simulink library "chyc_rebuild_chyc_20170830_std"  (R2012b)
settings: Solver=ode45  StartTime=0.0  StopTime=10.0  RelTol=1e-3
undefined symbols (not defined in the file): sMP
libraries: simulink x6, simulink_extras x1
settings Model: Creator=LAUEREL  LastModifiedBy=LAUEREL

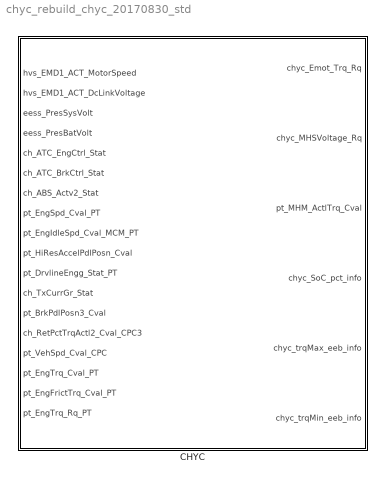
== system chyc_rebuild_chyc_20170830_std ==
  CHYC : Subsystem  mask(MapModule){chyc_EM_BstApp_DeltaEngSpd=sMP.ctrl.chyc.EM_BstApp_DeltaEngSpd, chyc_EM_BstApp_thresh_AccPedal=sMP.ctrl.chyc.EM_BstApp_thresh_AccPedal, chyc_EM_BstTrq_BrkPt_SoC=sMP.ctrl.chyc.EM_BstTrq_BrkPt_SoC, chyc_EM_BstTrq_BrkPt_VehSpd=sMP.ctrl.chyc.EM_BstTrq_BrkPt_VehSpd, chyc_EM_BstTrq_Map_BstTrq=sMP.ctrl.chyc.EM_BstTrq_Map_BstTrq, chyc_EM_BstTrq_TrqAuxSupport=sMP.ctrl.chyc.EM_BstTrq_TrqAuxSupport, chyc_EM_BstTrq_hyst_SoCforAuxSupport=sMP.ctrl.chyc.EM_BstTrq_hyst_SoCforAuxSupport, chyc_EM_BstTrq_thresh_GearforBoost=sMP.ctrl.chyc.EM_BstTrq_thresh_GearforBoost, chyc_EM_BstTrq_thresh_SoCforAuxSupport=sMP.ctrl.chyc.EM_BstTrq_thresh_SoCforAuxSupport, chyc_EM_ElBound_CurrMax=sMP.ctrl.chyc.EM_ElBound_CurrMax, chyc_EM_ElBound_CurrMin=sMP.ctrl.chyc.EM_ElBound_CurrMin, chyc_EM_ElBound_VltMax=sMP.ctrl.chyc.EM_ElBound_VltMax, chyc_EM_ElBound_VltMin=sMP.ctrl.chyc.EM_ElBound_VltMin, chyc_EM_ElBound_VltTarget=sMP.ctrl.chyc.EM_ElBound_VltTarget, chyc_EM_Fummel_TrqTargetLimit_boost=sMP.ctrl.chyc.EM_Fummel_TrqTargetLimit_boost, chyc_EM_Fummel_TrqTargetLimit_recup=sMP.ctrl.chyc.EM_Fummel_TrqTargetLimit_recup, chyc_EM_Fummel_rateDelay_ZeroCross_boost=sMP.ctrl.chyc.EM_Fummel_rateDelay_ZeroCross_boost, chyc_EM_Fummel_rateDelay_ZeroCross_recup=sMP.ctrl.chyc.EM_Fummel_rateDelay_ZeroCross_recup, chyc_EM_Fummel_trqRateLimit_ZeroCross_boost=sMP.ctrl.chyc.EM_Fummel_trqRateLimit_ZeroCross_boost, chyc_EM_Fummel_trqRateLimit_ZeroCross_recup=sMP.ctrl.chyc.EM_Fummel_trqRateLimit_ZeroCross_recup, chyc_EM_Fummel_trqRateLimit_boost=sMP.ctrl.chyc.EM_Fummel_trqRateLimit_boost, chyc_EM_Fummel_trqRateLimit_recup=sMP.ctrl.chyc.EM_Fummel_trqRateLimit_recup, chyc_EM_Fummel_trqThreshold_ZeroCross_boost=sMP.ctrl.chyc.EM_Fummel_trqThreshold_ZeroCross_boost, chyc_EM_Fummel_trqThreshold_ZeroCross_recup=sMP.ctrl.chyc.EM_Fummel_trqThreshold_ZeroCross_recup, chyc_EM_RecApp_thresh_GearforRecup=sMP.ctrl.chyc.EM_RecApp_thresh_GearforRecup, chyc_EM_RecApp_thresh_NoAccPedal=sMP.ctrl.chyc.EM_RecApp_thresh_NoAccPedal, chyc_EM_RecTrq_MaxRecTrq=sMP.ctrl.chyc.EM_RecTrq_MaxRecTrq, chyc_EM_RecTrq_PropFactor=sMP.ctrl.chyc.EM_RecTrq_PropFactor, chyc_EM_RecTrq_RWhl=sMP.ctrl.chyc.EM_RecTrq_RWhl, chyc_EM_RecTrq_RefWeight=sMP.ctrl.chyc.EM_RecTrq_RefWeight, chyc_EM_RecTrq_thresh_RetTrq=sMP.ctrl.chyc.EM_RecTrq_thresh_RetTrq, chyc_EM_TgtDet_EMTrqcutoff_abs=sMP.ctrl.chyc.EM_TgtDet_EMTrqcutoff_abs, chyc_EM_TgtDet_thresh_EngSpdAboveIdle=sMP.ctrl.chyc.EM_TgtDet_thresh_EngSpdAboveIdle, chyc_EM_TgtDet_thresh_EngTrqforRecup=sMP.ctrl.chyc.EM_TgtDet_thresh_EngTrqforRecup, chyc_EM_TgtDet_trqRateLimit_EBS_activate_neg=sMP.ctrl.chyc.EM_TgtDet_trqRateLimit_EBS_activate_neg, chyc_EM_TgtDet_trqRateLimit_EBS_activate_pos=sMP.ctrl.chyc.EM_TgtDet_trqRateLimit_EBS_activate_pos, chyc_EM_TgtDet_trqRateLimit_boost=sMP.ctrl.chyc.EM_TgtDet_trqRateLimit_boost, chyc_EM_TgtDet_trqRateLimit_recup=sMP.ctrl.chyc.EM_TgtDet_trqRateLimit_recup, chyc_EM_VersionNumber=sMP.ctrl.chyc.EM_VersionNumber, chyc_MHS_capacity=sMP.ctrl.chyc.MHS_capacity, chyc_MHS_U_cap_max=sMP.ctrl.chyc.MHS_U_cap_max, chyc_MHS_U_cap_min=sMP.ctrl.chyc.MHS_U_cap_min, chyc_MHS_nParallel=sMP.ctrl.chyc.MHS_nParallel, chyc_MHS_dcdc_Pmax_chg=sMP.ctrl.chyc.MHS_dcdc_Pmax_chg, chyc_MHS_dcdc_Pmax_dischg=sMP.ctrl.chyc.MHS_dcdc_Pmax_dischg, chyc_MHS_dcdc_U_Cap=sMP.ctrl.chyc.MHS_dcdc_U_Cap, chyc_MHS_dcdc_U_ZK=sMP.ctrl.chyc.MHS_dcdc_U_ZK, chyc_MHS_PEEBmax=sMP.ctrl.chyc.MHS_PEEBmax, chyc_mot_trqTab=sMP.ctrl.chyc.mot_trqTab, chyc_mot_nTab=sMP.ctrl.chyc.mot_nTab, chyc_mot_vltTab=sMP.ctrl.chyc.mot_vltTab, chyc_mot_Pmax_PTab=sMP.ctrl.chyc.mot_Pmax_PTab, chyc_mot_Pmax_PTab_trqTab=sMP.ctrl.chyc.mot_Pmax_PTab_trqTab, chyc_mot_eng_Pmax_HiLS=sMP.ctrl.chyc.mot_eng_Pmax_HiLS, chyc_mot_trqMax_vltTab=sMP.ctrl.chyc.mot_trqMax_vltTab, chyc_mot_trqMax_nTab=sMP.ctrl.chyc.mot_trqMax_nTab, chyc_mot_trqMax_trqTab_peak=sMP.ctrl.chyc.mot_trqMax_trqTab_peak, chyc_mot_trqMin_vltTab=sMP.ctrl.chyc.mot_trqMin_vltTab, chyc_mot_trqMin_nTab=sMP.ctrl.chyc.mot_trqMin_nTab, chyc_mot_trqMin_trqTab_peak=sMP.ctrl.chyc.mot_trqMin_trqTab_peak}

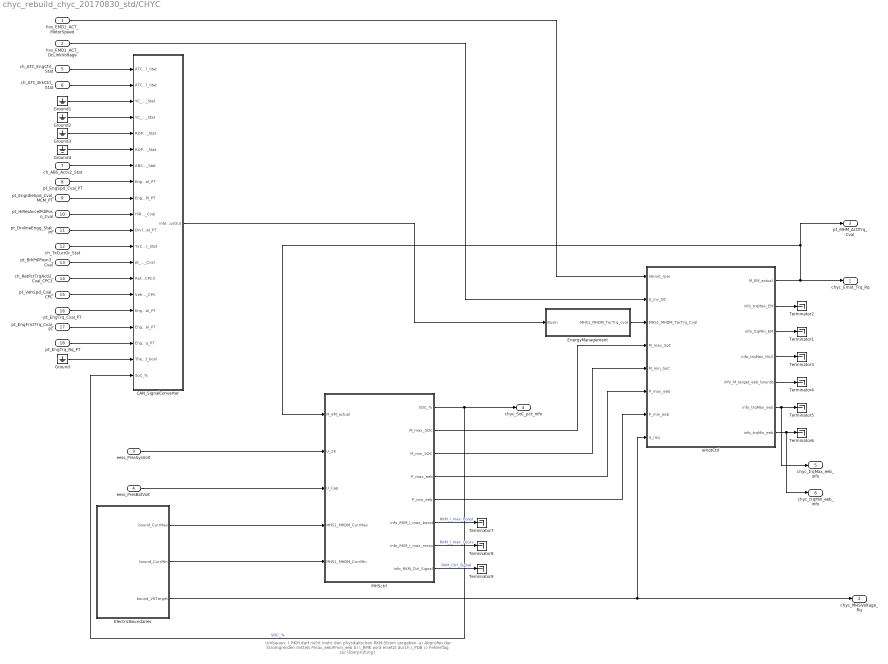
== system chyc_rebuild_chyc_20170830_std/CHYC ==
  note: Umbauen: I_RKM darf nicht mehr den physikalischen RKM-Strom vorgeben.
      | a) Abprüfen der Stromgrenzen mittels Pmax_eeb/Pmin_eeb
      | b) I_RMK wird ersetzt durch I_PDB
      | c) Fehlerflag zur Überprüfung?
  hvs_EMD1_ACT_MotorSpeed : Inport
  hvs_EMD1_ACT_DcLinkVoltage : Inport  Port=2
  eess_PresSysVolt : Inport  Port=3
  eess_PresBatVolt : Inport  Port=4
  ch_ATC_EngCtrl_Stat : Inport  Port=5
  ch_ATC_BrkCtrl_Stat : Inport  Port=6
  ch_ABS_Actv2_Stat : Inport  Port=7
  pt_EngSpd_Cval_PT : Inport  Port=8
  pt_EngIdleSpd_Cval_MCM_PT : Inport  Port=9
  pt_HiResAccelPdlPosn_Cval : Inport  Port=10
  pt_DrvlineEngg_Stat_PT : Inport  Port=11
  ch_TxCurrGr_Stat : Inport  Port=12
  pt_BrkPdlPosn3_Cval : Inport  Port=13
  ch_RetPctTrqActl2_Cval_CPC3 : Inport  Port=14
  pt_VehSpd_Cval_CPC : Inport  Port=15
  pt_EngTrq_Cval_PT : Inport  Port=16
  pt_EngFrictTrq_Cval_PT : Inport  Port=17
  pt_EngTrq_Rq_PT : Inport  Port=18
  CAN_SignalConverter : Subsystem
  ElectricBoundaries : Subsystem
  EnergyManagement : Subsystem
  Ground{,1..4} (5 alike) : Ground
  MHSctrl : Subsystem
  Terminator{1..9} (9 alike) : Terminator
  emotCtrl : Subsystem
  chyc_Emot_Trq_Rq : Outport
  chyc_MHSVoltage_Rq : Outport  Port=2
  pt_MHM_ActlTrq_Cval : Outport  Port=3
  chyc_SoC_pct_info : Outport  Port=4
  chyc_trqMax_eeb_info : Outport  Port=5
  chyc_trqMin_eeb_info : Outport  Port=6
  wires:
  EnergyManagement/1(MHS1_MHDM_TarTrq_cval) -> emotCtrl/3(MHS1_MHDM_TarTrq_Cval)
  CAN_SignalConverter/1(internalBusOut) -> EnergyManagement/1(BusIn)
  emotCtrl/2(info_trqMax_EM) -> Terminator2/1
  emotCtrl/3(info_trqMin_EM) -> Terminator1/1
  emotCtrl/4(info_trqMax_HiLS) -> Terminator3/1
  emotCtrl/5(info_M_target_eeb_bounds) -> Terminator4/1
  emotCtrl/6(info_trqMax_eeb) -> chyc_trqMax_eeb_info/1, Terminator5/1
  emotCtrl/7(info_trqMin_eeb) -> chyc_trqMin_eeb_info/1, Terminator6/1
  emotCtrl/1(M_EM_actual) -> chyc_Emot_Trq_Rq/1, pt_MHM_ActlTrq_Cval/1, MHSctrl/1(M_EM_actual)
  eess_PresSysVolt/1 -> MHSctrl/2(U_ZK)
  eess_PresBatVolt/1 -> MHSctrl/3(U_Cap)
  MHSctrl/3(M_min_SOC) -> emotCtrl/5(M_min_SoC)
  MHSctrl/2(M_max_SOC) -> emotCtrl/4(M_max_SoC)
  MHSctrl/1(SOC_%) -> CAN_SignalConverter/20(SoC_%), chyc_SoC_pct_info/1  "SOC_%"
  ElectricBoundaries/3(bound_VltTarget) -> chyc_MHSVoltage_Rq/1, emotCtrl/8(U_req)
  ElectricBoundaries/1(bound_CurrMax) -> MHSctrl/4(MHS1_MHDM_CurrMax)
  ElectricBoundaries/2(bound_CurrMin) -> MHSctrl/5(MHS1_MHDM_CurrMin)
  MHSctrl/6(info_RKM_I_max_boost) -> Terminator7/1  "RKM_I_max_boost"
  MHSctrl/7(info_RKM_I_max_recov) -> Terminator8/1  "RKM_I_max_recov"
  MHSctrl/8(info_RKM_Ctrl_Signal) -> Terminator9/1  "RKM_Ctrl_Signal"
  hvs_EMD1_ACT_MotorSpeed/1 -> emotCtrl/1(nEmot_rpm)
  MHSctrl/5(P_min_eeb) -> emotCtrl/7(P_min_eeb)
  MHSctrl/4(P_max_eeb) -> emotCtrl/6(P_max_eeb)
  hvs_EMD1_ACT_DcLinkVoltage/1 -> emotCtrl/2(U_inv_DC)
  Ground4/1 -> CAN_SignalConverter/6(ROP_EngCtrlActv2_Stat)
  pt_BrkPdlPosn3_Cval/1 -> CAN_SignalConverter/13(pt_BrkPdlPosn3_Cval)
  pt_EngTrq_Rq_PT/1 -> CAN_SignalConverter/18(EngTrqRq_PT)
  pt_EngSpd_Cval_PT/1 -> CAN_SignalConverter/8(EngSpd_Cval_PT)
  pt_HiResAccelPdlPosn_Cval/1 -> CAN_SignalConverter/10(HiResAccelPosn_Cval)
  pt_EngFrictTrq_Cval_PT/1 -> CAN_SignalConverter/17(EngFricTrq_Cval_PT)
  ch_ATC_BrkCtrl_Stat/1 -> CAN_SignalConverter/2(ATC_BrkCtrl_Stat)
  ch_ATC_EngCtrl_Stat/1 -> CAN_SignalConverter/1(ATC_EngCtrl_Stat)
  ch_RetPctTrqActl2_Cval_CPC3/1 -> CAN_SignalConverter/14(RetPctTrqActl2_Cval_CPC3)
  pt_VehSpd_Cval_CPC/1 -> CAN_SignalConverter/15(VehSpd_Cval_CPC)
  pt_EngTrq_Cval_PT/1 -> CAN_SignalConverter/16(EngTrq_Cval_PT)
  Ground3/1 -> CAN_SignalConverter/5(ROP_BrkCtrlActv2_Stat)
  ch_TxCurrGr_Stat/1 -> CAN_SignalConverter/12(TxCurrGr_Stat)
  ch_ABS_Actv2_Stat/1 -> CAN_SignalConverter/7(ABS_Actv_Stat)
  Ground2/1 -> CAN_SignalConverter/4(YC_EngCtrlActv2_Stat)
  Ground/1 -> CAN_SignalConverter/19(ThermoSupport_bool)
  pt_DrvlineEngg_Stat_PT/1 -> CAN_SignalConverter/11(DrvlineEngg_Stat_PT)
  pt_EngIdleSpd_Cval_MCM_PT/1 -> CAN_SignalConverter/9(EngIdleSpd_Cval_MCM_PT)
  Ground1/1 -> CAN_SignalConverter/3(YC_BrkCtrlActv2_Stat)

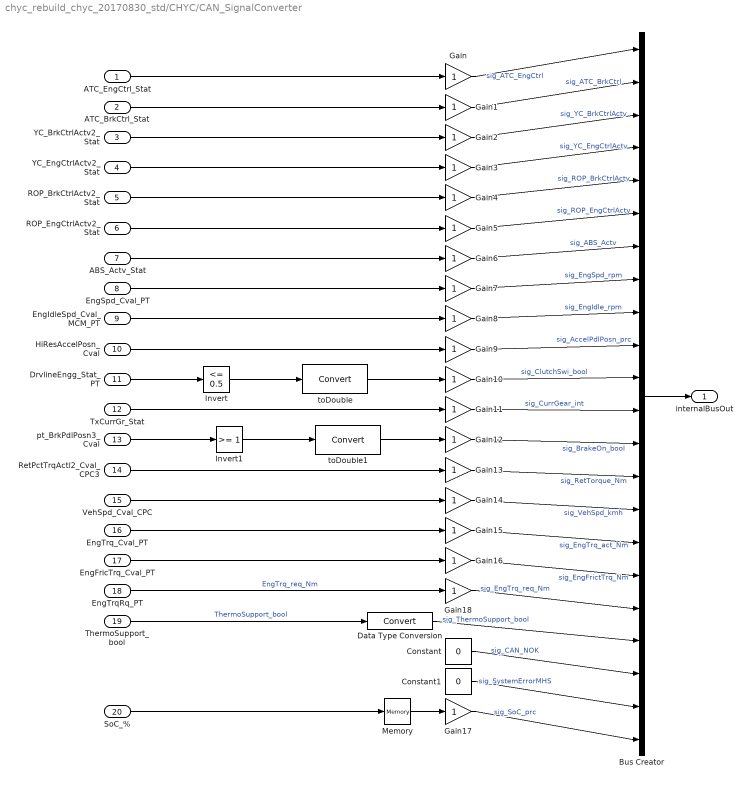
== system chyc_rebuild_chyc_20170830_std/CHYC/CAN_SignalConverter ==
  ATC_EngCtrl_Stat : Inport
  ATC_BrkCtrl_Stat : Inport  Port=2
  YC_BrkCtrlActv2_Stat : Inport  Port=3
  YC_EngCtrlActv2_Stat : Inport  Port=4
  ROP_BrkCtrlActv2_Stat : Inport  Port=5
  ROP_EngCtrlActv2_Stat : Inport  Port=6
  ABS_Actv_Stat : Inport  Port=7
  EngSpd_Cval_PT : Inport  Port=8
  EngIdleSpd_Cval_MCM_PT : Inport  Port=9
  HiResAccelPosn_Cval : Inport  Port=10
  DrvlineEngg_Stat_PT : Inport  Port=11
  TxCurrGr_Stat : Inport  Port=12
  pt_BrkPdlPosn3_Cval : Inport  Port=13
  RetPctTrqActl2_Cval_CPC3 : Inport  Port=14
  VehSpd_Cval_CPC : Inport  Port=15
  EngTrq_Cval_PT : Inport  Port=16
  EngFricTrq_Cval_PT : Inport  Port=17
  EngTrqRq_PT : Inport  Port=18
  ThermoSupport_bool : Inport  Port=19
  SoC_% : Inport  Port=20
  Bus Creator : BusCreator  Inputs=22
  Constant : Constant  Value=0
  Constant1 : Constant  Value=0
  Data Type Conversion : DataTypeConversion
  Gain{,1..18} (19 alike) : Gain
  Invert : simulink/Logic and Bit Operations/Compare To Constant  relop=<=  const=0.5  OutDataTypeStr=boolean
  Invert1 : simulink/Logic and Bit Operations/Compare To Constant  relop=>=  const=1  OutDataTypeStr=boolean
  Memory : Memory
  toDouble : DataTypeConversion
  toDouble1 : DataTypeConversion
  internalBusOut : Outport
  wires:
  SoC_%/1 -> Memory/1
  Gain/1 -> Bus Creator/1  "sig_ATC_EngCtrl"
  Gain1/1 -> Bus Creator/2  "sig_ATC_BrkCtrl"
  Gain2/1 -> Bus Creator/3  "sig_YC_BrkCtrlActv"
  Gain3/1 -> Bus Creator/4  "sig_YC_EngCtrlActv"
  Gain4/1 -> Bus Creator/5  "sig_ROP_BrkCtrlActv"
  Gain5/1 -> Bus Creator/6  "sig_ROP_EngCtrlActv"
  Gain9/1 -> Bus Creator/10  "sig_AccelPdlPosn_prc"
  Gain6/1 -> Bus Creator/7  "sig_ABS_Actv"
  Gain7/1 -> Bus Creator/8  "sig_EngSpd_rpm"
  Gain10/1 -> Bus Creator/11  "sig_ClutchSwi_bool"
  Gain8/1 -> Bus Creator/9  "sig_EngIdle_rpm"
  Gain11/1 -> Bus Creator/12  "sig_CurrGear_int"
  Gain12/1 -> Bus Creator/13  "sig_BrakeOn_bool"
  Gain13/1 -> Bus Creator/14  "sig_RetTorque_Nm"
  Gain15/1 -> Bus Creator/16  "sig_EngTrq_act_Nm"
  Gain14/1 -> Bus Creator/15  "sig_VehSpd_kmh"
  Gain17/1 -> Bus Creator/22  "sig_SoC_prc"
  Gain16/1 -> Bus Creator/17  "sig_EngFrictTrq_Nm"
  Data Type Conversion/1 -> Bus Creator/19  "sig_ThermoSupport_bool"
  Gain18/1 -> Bus Creator/18  "sig_EngTrq_req_Nm"
  Memory/1 -> Gain17/1
  Bus Creator/1 -> internalBusOut/1
  Constant/1 -> Bus Creator/20  "sig_CAN_NOK"
  Constant1/1 -> Bus Creator/21  "sig_SystemErrorMHS"
  TxCurrGr_Stat/1 -> Gain11/1
  EngFricTrq_Cval_PT/1 -> Gain16/1
  VehSpd_Cval_CPC/1 -> Gain14/1
  RetPctTrqActl2_Cval_CPC3/1 -> Gain13/1
  EngTrq_Cval_PT/1 -> Gain15/1
  Invert/1 -> toDouble/1
  HiResAccelPosn_Cval/1 -> Gain9/1
  EngIdleSpd_Cval_MCM_PT/1 -> Gain8/1
  ABS_Actv_Stat/1 -> Gain6/1
  ROP_EngCtrlActv2_Stat/1 -> Gain5/1
  ROP_BrkCtrlActv2_Stat/1 -> Gain4/1
  YC_EngCtrlActv2_Stat/1 -> Gain3/1
  YC_BrkCtrlActv2_Stat/1 -> Gain2/1
  ATC_BrkCtrl_Stat/1 -> Gain1/1
  ATC_EngCtrl_Stat/1 -> Gain/1
  EngSpd_Cval_PT/1 -> Gain7/1
  EngTrqRq_PT/1 -> Gain18/1  "EngTrq_req_Nm"
  ThermoSupport_bool/1 -> Data Type Conversion/1  "ThermoSupport_bool"
  DrvlineEngg_Stat_PT/1 -> Invert/1
  toDouble/1 -> Gain10/1
  Invert1/1 -> toDouble1/1
  toDouble1/1 -> Gain12/1
  pt_BrkPdlPosn3_Cval/1 -> Invert1/1

== system chyc_rebuild_chyc_20170830_std/CHYC/ElectricBoundaries ==
  CurrMax : Constant  Value=chyc_EM_ElBound_CurrMax
  CurrMin : Constant  Value=chyc_EM_ElBound_CurrMin
  VltTarget : Constant  Value=chyc_EM_ElBound_VltTarget
  bound_CurrMax : Outport
  bound_CurrMin : Outport  Port=2
  bound_VltTarget : Outport  Port=3
  wires:
  CurrMax/1 -> bound_CurrMax/1  "MHS1_MHDM_CurrMax_cval"
  CurrMin/1 -> bound_CurrMin/1  "MHS1_MHDM_CurrMin_cval"
  VltTarget/1 -> bound_VltTarget/1  "MHS1_MHDM_VltTarget"

== system chyc_rebuild_chyc_20170830_std/CHYC/EnergyManagement ==
  BusIn : Inport
  BoostApproval : Subsystem
  BoostTorque : Subsystem
  NoEBSFunction : Subsystem
  RecuperationApproval : Subsystem
  RecuperationTorque : Subsystem
  TargetDetermination : Subsystem
  MHS1_MHDM_TarTrq_cval : Outport
  wires:
  NoEBSFunction/1(NoEBSFunction) -> TargetDetermination/1(NoEBSFunction)
  TargetDetermination/1(MHS1_MHDM_TarTrq_cval) -> MHS1_MHDM_TarTrq_cval/1
  RecuperationApproval/1(RecApproved) -> TargetDetermination/2(RecApproved)
  BoostApproval/1(BoostApproved) -> TargetDetermination/3(BoostApproved)
  RecuperationTorque/1(TargetRecuperation) -> TargetDetermination/4(TargetRecuperation)
  BoostTorque/1(TargetBoost) -> TargetDetermination/5(TargetBoost)
  BusIn/1 -> BoostTorque/1(BusIn), TargetDetermination/6(BusIn), RecuperationTorque/1(BusIn), BoostApproval/1(BusIn), RecuperationApproval/1(BusIn), NoEBSFunction/1(BusIn)  "ClutchSwTop_Rq"

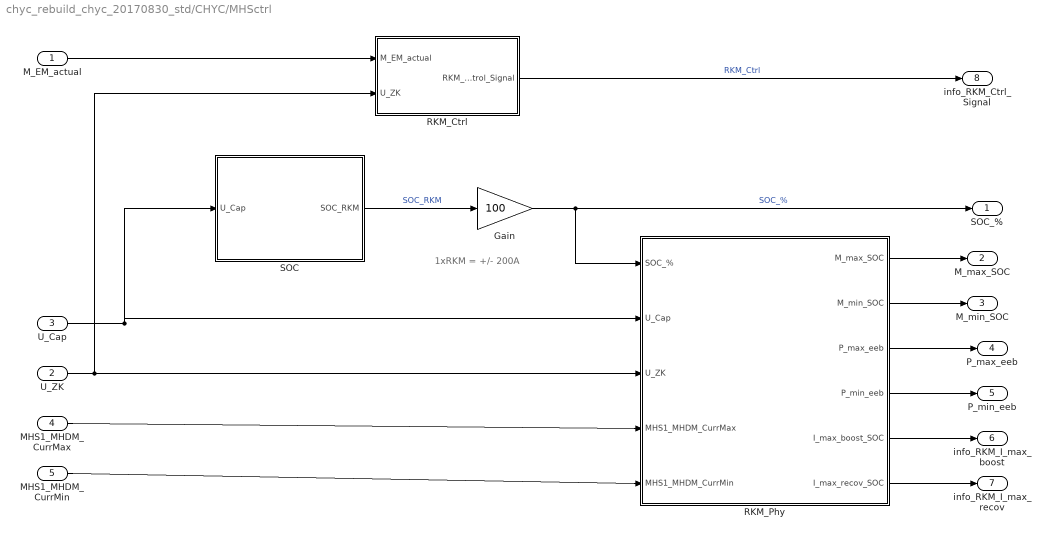
== system chyc_rebuild_chyc_20170830_std/CHYC/MHSctrl ==
  note: 1xRKM = +/- 200A
  M_EM_actual : Inport
  U_ZK : Inport  Port=2
  U_Cap : Inport  Port=3
  MHS1_MHDM_CurrMax : Inport  Port=4
  MHS1_MHDM_CurrMin : Inport  Port=5
  Gain : Gain  Gain=100
  "RKM_Ctrl " : Subsystem
  RKM_Phy : Subsystem
  SOC : Subsystem
  SOC_% : Outport  InitialOutput=0
  M_max_SOC : Outport  Port=2
  M_min_SOC : Outport  Port=3
  P_max_eeb : Outport  Port=4
  P_min_eeb : Outport  Port=5
  info_RKM_I_max_boost : Outport  Port=6
  info_RKM_I_max_recov : Outport  Port=7
  info_RKM_Ctrl_Signal : Outport  Port=8
  wires:
  RKM_Phy/4(P_min_eeb) -> P_min_eeb/1
  RKM_Phy/3(P_max_eeb) -> P_max_eeb/1
  RKM_Phy/2(M_min_SOC) -> M_min_SOC/1
  RKM_Phy/1(M_max_SOC) -> M_max_SOC/1
  RKM_Phy/6(I_max_recov_SOC) -> info_RKM_I_max_recov/1
  RKM_Phy/5(I_max_boost_SOC) -> info_RKM_I_max_boost/1
  Gain/1 -> RKM_Phy/1(SOC_%), SOC_%/1  "SOC_%"
  SOC/1(SOC_RKM) -> Gain/1  "SOC_RKM"
  U_Cap/1 -> SOC/1(U_Cap), RKM_Phy/2(U_Cap)
  U_ZK/1 -> RKM_Phy/3(U_ZK), "RKM_Ctrl "/2("U_ZK ")
  M_EM_actual/1 -> "RKM_Ctrl "/1(M_EM_actual)
  "RKM_Ctrl "/1(RKM_Control_Signal) -> info_RKM_Ctrl_Signal/1  "RKM_Ctrl"
  MHS1_MHDM_CurrMax/1 -> RKM_Phy/4(MHS1_MHDM_CurrMax)
  MHS1_MHDM_CurrMin/1 -> RKM_Phy/5(MHS1_MHDM_CurrMin)

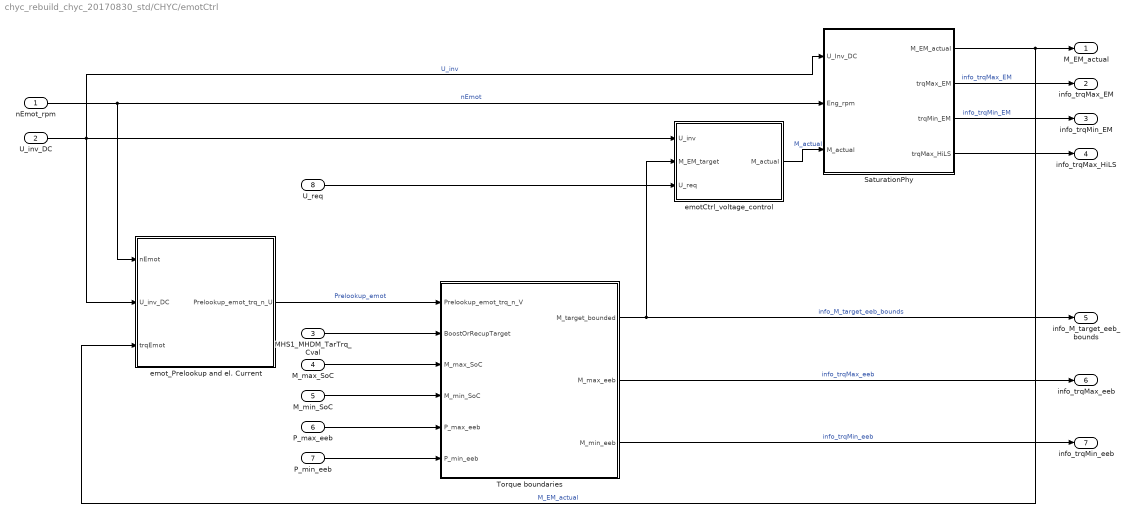
== system chyc_rebuild_chyc_20170830_std/CHYC/emotCtrl ==
  nEmot_rpm : Inport
  U_inv_DC : Inport  Port=2
  MHS1_MHDM_TarTrq_Cval : Inport  Port=3
  M_max_SoC : Inport  Port=4
  M_min_SoC : Inport  Port=5
  P_max_eeb : Inport  Port=6
  P_min_eeb : Inport  Port=7
  U_req : Inport  Port=8
  SaturationPhy : Subsystem
  Torque boundaries : Subsystem
  emotCtrl_voltage_control : Subsystem
  emot_Prelookup and el. Current : Subsystem
  M_EM_actual : Outport
  info_trqMax_EM : Outport  Port=2
  info_trqMin_EM : Outport  Port=3
  info_trqMax_HiLS : Outport  Port=4
  info_M_target_eeb_bounds : Outport  Port=5
  info_trqMax_eeb : Outport  Port=6
  info_trqMin_eeb : Outport  Port=7
  wires:
  SaturationPhy/1(M_EM_actual) -> emot_Prelookup and el. Current/3(trqEmot), M_EM_actual/1  "M_EM_actual"
  nEmot_rpm/1 -> emot_Prelookup and el. Current/1(nEmot), SaturationPhy/2(Eng_rpm)  "nEmot"
  U_inv_DC/1 -> emot_Prelookup and el. Current/2(U_inv_DC), SaturationPhy/1(U_Inv_DC), emotCtrl_voltage_control/1(U_inv)  "U_inv"
  MHS1_MHDM_TarTrq_Cval/1 -> Torque boundaries/2(BoostOrRecupTarget)
  emotCtrl_voltage_control/1(M_actual) -> SaturationPhy/3(M_actual)  "M_actual"
  SaturationPhy/2(trqMax_EM) -> info_trqMax_EM/1  "info_trqMax_EM"
  SaturationPhy/3(trqMin_EM) -> info_trqMin_EM/1  "info_trqMin_EM"
  SaturationPhy/4(trqMax_HiLS) -> info_trqMax_HiLS/1
  P_max_eeb/1 -> Torque boundaries/5(P_max_eeb)
  M_max_SoC/1 -> Torque boundaries/3(M_max_SoC)
  M_min_SoC/1 -> Torque boundaries/4(M_min_SoC)
  P_min_eeb/1 -> Torque boundaries/6(P_min_eeb)
  Torque boundaries/1(M_target_bounded) -> info_M_target_eeb_bounds/1, emotCtrl_voltage_control/2(M_EM_target)  "info_M_target_eeb_bounds"
  Torque boundaries/2(M_max_eeb) -> info_trqMax_eeb/1  "info_trqMax_eeb"
  Torque boundaries/3(M_min_eeb) -> info_trqMin_eeb/1  "info_trqMin_eeb"
  U_req/1 -> emotCtrl_voltage_control/3(U_req)
  emot_Prelookup and el. Current/1(Prelookup_emot_trq_n_U) -> Torque boundaries/1(Prelookup_emot_trq_n_V)  "Prelookup_emot"

== system chyc_rebuild_chyc_20170830_std/CHYC/EnergyManagement/BoostApproval ==
  BusIn : Inport
  Accpdl : RelationalOperator  Operator=>  OutDataTypeStr=boolean
  Add : Sum
  Bus Selector2 : BusSelector  OutputSignals=sig_ThermoSupport_bool,sig_AccelPdlPosn_prc,sig_EngSpd_rpm,sig_EngIdle_rpm
  Constant1 : Constant  Value=chyc_EM_BstApp_thresh_AccPedal  OutDataTypeStr=uint16
  Constant2 : Constant  Value=0  OutDataTypeStr=uint16
  Logical Operator : Logic  AllPortsSameDT=off  OutDataTypeStr=boolean
  Logical Operator1 : Logic  Operator=OR  AllPortsSameDT=off  OutDataTypeStr=boolean
  NoDriveoffPossible : RelationalOperator  Operator=<  OutDataTypeStr=boolean
  NoThermoSupport : RelationalOperator  Operator===  OutDataTypeStr=boolean
  offset rpm : Constant  Value=chyc_EM_BstApp_DeltaEngSpd
  BoostApproved : Outport
  wires:
  NoThermoSupport/1 -> Logical Operator/1  "sig_NoThermoSupport"
  Constant2/1 -> NoThermoSupport/2
  Accpdl/1 -> Logical Operator1/1
  Logical Operator1/1 -> Logical Operator/2  "sig_TractionStateOrIdle"
  Constant1/1 -> Accpdl/2
  Logical Operator/1 -> BoostApproved/1  "sig_BoostApproved"
  NoDriveoffPossible/1 -> Logical Operator1/2
  Add/1 -> NoDriveoffPossible/2
  offset rpm/1 -> Add/2
  Bus Selector2/4 -> Add/1  "<sig_EngIdle_rpm>"
  BusIn/1 -> Bus Selector2/1  "ClutchSwTop_Rq"
  Bus Selector2/3 -> NoDriveoffPossible/1  "<sig_EngSpd_rpm>"
  Bus Selector2/1 -> NoThermoSupport/1  "<sig_ThermoSupport_bool>"
  Bus Selector2/2 -> Accpdl/1  "<sig_AccelPdlPosn_prc>"

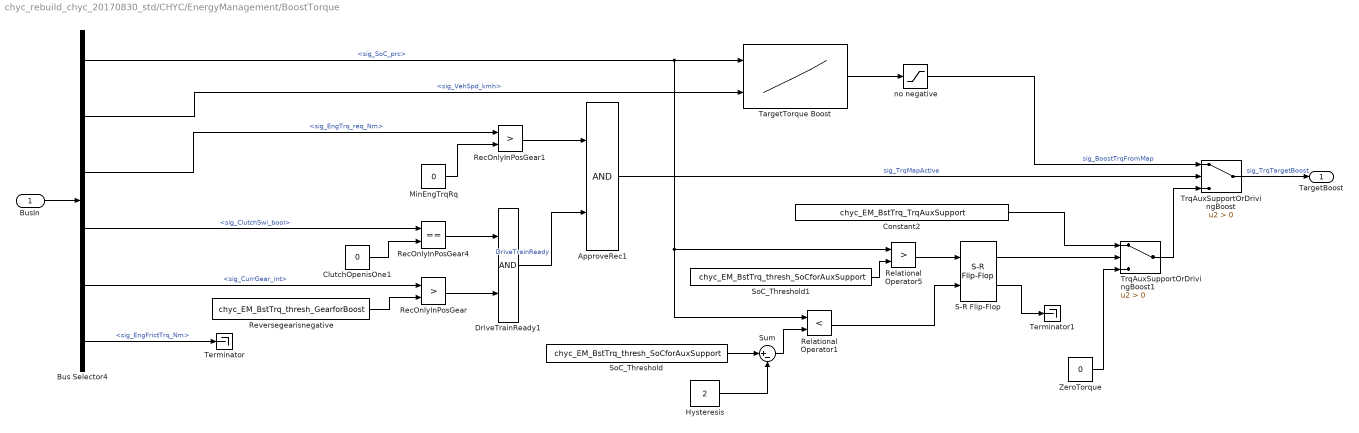
== system chyc_rebuild_chyc_20170830_std/CHYC/EnergyManagement/BoostTorque ==
  BusIn : Inport
  ApproveRec1 : Logic  AllPortsSameDT=off  OutDataTypeStr=boolean
  Bus Selector4 : BusSelector  OutputSignals=sig_SoC_prc,sig_VehSpd_kmh,sig_EngTrq_req_Nm,sig_ClutchSwi_bool,sig_CurrGear_int,sig_EngFrictTrq_Nm
  ClutchOpenisOne1 : Constant  Value=0
  Constant2 : Constant  Value=chyc_EM_BstTrq_TrqAuxSupport
  DriveTrainReady1 : Logic  AllPortsSameDT=off  OutDataTypeStr=boolean
  Hysteresis : Constant  Value=2
  MinEngTrqRq : Constant  Value=0
  RecOnlyInPosGear : RelationalOperator  Operator=>  OutDataTypeStr=boolean
  RecOnlyInPosGear1 : RelationalOperator  Operator=>  OutDataTypeStr=boolean
  RecOnlyInPosGear4 : RelationalOperator  Operator===  OutDataTypeStr=boolean
  Relational Operator1 : RelationalOperator  Operator=<  OutDataTypeStr=boolean
  Relational Operator5 : RelationalOperator  Operator=>  OutDataTypeStr=boolean
  Reversegearisnegative : Constant  Value=chyc_EM_BstTrq_thresh_GearforBoost  VectorParams1D=off
  S-R Flip-Flop : simulink_extras/Flip Flops/S-R Flip-Flop  initial_condition=0
  SoC_Threshold : Constant  Value=chyc_EM_BstTrq_thresh_SoCforAuxSupport
  SoC_Threshold1 : Constant  Value=chyc_EM_BstTrq_thresh_SoCforAuxSupport
  Sum : Sum  Inputs=|+-
  TargetTorque Boost : Lookup_n-D  BreakpointsForDimension1=chyc_EM_BstTrq_BrkPt_SoC  BreakpointsForDimension2=chyc_EM_BstTrq_BrkPt_VehSpd  Table=chyc_EM_BstTrq_Map_BstTrq  ExtrapMethod=Clip  UseLastTableValue=on  RndMeth=Simplest  InputSameDT=on
  Terminator : Terminator
  Terminator1 : Terminator
  TrqAuxSupportOrDrivingBoost : Switch  Criteria=u2 > Threshold
  TrqAuxSupportOrDrivingBoost1 : Switch  Criteria=u2 > Threshold
  ZeroTorque : Constant  Value=0
  no negative : Saturate  UpperLimit=inf  LowerLimit=0
  TargetBoost : Outport
  wires:
  TrqAuxSupportOrDrivingBoost1/1 -> TrqAuxSupportOrDrivingBoost/3
  ZeroTorque/1 -> TrqAuxSupportOrDrivingBoost1/3
  S-R Flip-Flop/2 -> Terminator1/1
  S-R Flip-Flop/1 -> TrqAuxSupportOrDrivingBoost1/2
  Relational Operator1/1 -> S-R Flip-Flop/2
  Sum/1 -> Relational Operator1/2
  Hysteresis/1 -> Sum/2
  SoC_Threshold/1 -> Sum/1
  RecOnlyInPosGear1/1 -> ApproveRec1/1
  no negative/1 -> TrqAuxSupportOrDrivingBoost/1  "sig_BoostTrqFromMap"
  TrqAuxSupportOrDrivingBoost/1 -> TargetBoost/1  "sig_TrqTargetBoost"
  SoC_Threshold1/1 -> Relational Operator5/2
  ApproveRec1/1 -> TrqAuxSupportOrDrivingBoost/2  "sig_TrqMapActive"
  TargetTorque Boost/1 -> no negative/1
  Constant2/1 -> TrqAuxSupportOrDrivingBoost1/1
  Relational Operator5/1 -> S-R Flip-Flop/1
  Reversegearisnegative/1 -> RecOnlyInPosGear/2
  RecOnlyInPosGear/1 -> DriveTrainReady1/2
  ClutchOpenisOne1/1 -> RecOnlyInPosGear4/2
  RecOnlyInPosGear4/1 -> DriveTrainReady1/1
  DriveTrainReady1/1 -> ApproveRec1/2  "DriveTrainReady"
  MinEngTrqRq/1 -> RecOnlyInPosGear1/2
  BusIn/1 -> Bus Selector4/1
  Bus Selector4/2 -> TargetTorque Boost/2  "<sig_VehSpd_kmh>"
  Bus Selector4/6 -> Terminator/1  "<sig_EngFrictTrq_Nm>"
  Bus Selector4/5 -> RecOnlyInPosGear/1  "<sig_CurrGear_int>"
  Bus Selector4/4 -> RecOnlyInPosGear4/1  "<sig_ClutchSwi_bool>"
  Bus Selector4/1 -> Relational Operator1/1, Relational Operator5/1, TargetTorque Boost/1  "<sig_SoC_prc>"
  Bus Selector4/3 -> RecOnlyInPosGear1/1  "<sig_EngTrq_req_Nm>"

== system chyc_rebuild_chyc_20170830_std/CHYC/EnergyManagement/NoEBSFunction ==
  BusIn : Inport
  ApproveRec : Logic  Operator=NOR  Inputs=9  AllPortsSameDT=off  OutDataTypeStr=boolean
  Bus Selector : BusSelector  OutputSignals=sig_ATC_EngCtrl,sig_ATC_BrkCtrl,sig_YC_BrkCtrlActv,sig_YC_EngCtrlActv,sig_ROP_BrkCtrlActv,sig_ROP_EngCtrlActv,sig_ABS_Actv,sig_CAN_NOK,sig_SystemErrorMHS
  NoEBSFunction : Outport
  wires:
  ApproveRec/1 -> NoEBSFunction/1  "sig_NoEBSFunction"
  Bus Selector/7 -> ApproveRec/7  "<sig_ABS_Actv>"
  Bus Selector/6 -> ApproveRec/6  "<sig_ROP_EngCtrlActv>"
  Bus Selector/5 -> ApproveRec/5  "<sig_ROP_BrkCtrlActv>"
  Bus Selector/4 -> ApproveRec/4  "<sig_YC_EngCtrlActv>"
  Bus Selector/1 -> ApproveRec/1  "<sig_ATC_EngCtrl>"
  Bus Selector/3 -> ApproveRec/3  "<sig_YC_BrkCtrlActv>"
  Bus Selector/2 -> ApproveRec/2  "<sig_ATC_BrkCtrl>"
  BusIn/1 -> Bus Selector/1  "ClutchSwTop_Rq"
  Bus Selector/8 -> ApproveRec/8  "<sig_CAN_NOK>"
  Bus Selector/9 -> ApproveRec/9  "<sig_SystemErrorMHS>"

== system chyc_rebuild_chyc_20170830_std/CHYC/EnergyManagement/RecuperationApproval ==
  BusIn : Inport
  ApproveRec : Logic  AllPortsSameDT=off  OutDataTypeStr=boolean
  Bus Selector1 : BusSelector  OutputSignals=sig_AccelPdlPosn_prc,sig_ClutchSwi_bool,sig_CurrGear_int
  ClutchNotOpen : RelationalOperator  Operator===  OutDataTypeStr=boolean
  ClutchOpenisOne : Constant  Value=0
  DriveTrainReady : Logic  AllPortsSameDT=off  OutDataTypeStr=boolean
  No AccPedal : RelationalOperator  Operator===  OutDataTypeStr=boolean
  RecOnlyInPosGear : RelationalOperator  Operator=>  OutDataTypeStr=boolean
  Reversegearisnegative : Constant  Value=chyc_EM_RecApp_thresh_GearforRecup
  par_EM_RecApp_thresh_NoAccPedal : Constant  Value=chyc_EM_RecApp_thresh_NoAccPedal
  RecApproved : Outport
  wires:
  Reversegearisnegative/1 -> RecOnlyInPosGear/2
  RecOnlyInPosGear/1 -> DriveTrainReady/2
  Bus Selector1/2 -> ClutchNotOpen/1  "<sig_ClutchSwi_bool>"
  ApproveRec/1 -> RecApproved/1  "sig_RecApproved"
  Bus Selector1/1 -> No AccPedal/1  "<sig_AccelPdlPosn_prc>"
  par_EM_RecApp_thresh_NoAccPedal/1 -> No AccPedal/2
  No AccPedal/1 -> ApproveRec/1  "NoAccPdl"
  ClutchOpenisOne/1 -> ClutchNotOpen/2
  ClutchNotOpen/1 -> DriveTrainReady/1
  DriveTrainReady/1 -> ApproveRec/2  "sig_DriveTrainReady"
  BusIn/1 -> Bus Selector1/1
  Bus Selector1/3 -> RecOnlyInPosGear/1  "<sig_CurrGear_int>"

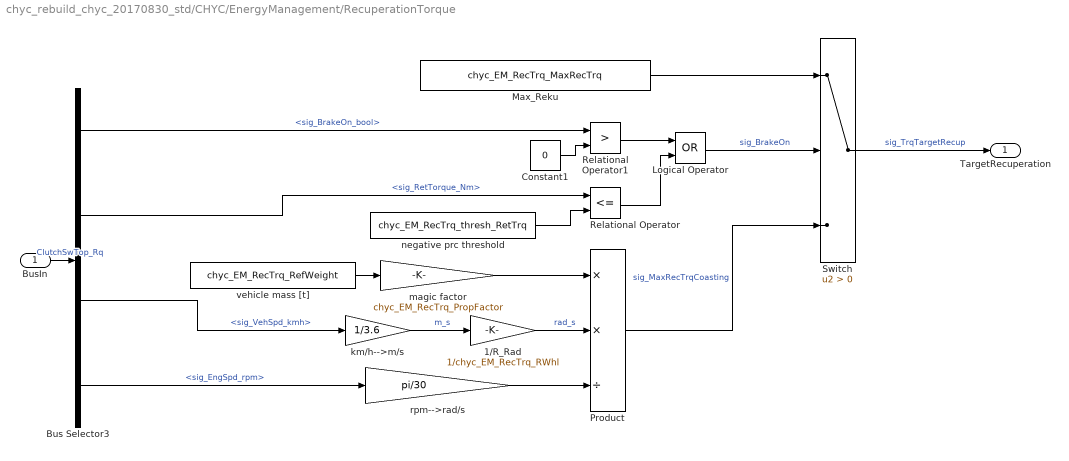
== system chyc_rebuild_chyc_20170830_std/CHYC/EnergyManagement/RecuperationTorque ==
  BusIn : Inport
  1/R_Rad : Gain  Gain=1/chyc_EM_RecTrq_RWhl
  Bus Selector3 : BusSelector  OutputSignals=sig_BrakeOn_bool,sig_RetTorque_Nm,sig_VehSpd_kmh,sig_EngSpd_rpm
  Constant1 : Constant  Value=0
  Logical Operator : Logic  Operator=OR  AllPortsSameDT=off  OutDataTypeStr=boolean
  Max_Reku : Constant  Value=chyc_EM_RecTrq_MaxRecTrq
  Product : Product  Inputs=**/  RndMeth=Zero
  Relational Operator : RelationalOperator  Operator=<=  OutDataTypeStr=boolean
  Relational Operator1 : RelationalOperator  Operator=>  OutDataTypeStr=boolean
  Switch : Switch  Criteria=u2 > Threshold
  km/h-->m/s : Gain  Gain=1/3.6
  magic factor : Gain  Gain=chyc_EM_RecTrq_PropFactor
  negative prc threshold : Constant  Value=chyc_EM_RecTrq_thresh_RetTrq
  rpm-->rad/s : Gain  Gain=pi/30
  vehicle mass [t] : Constant  Value=chyc_EM_RecTrq_RefWeight
  TargetRecuperation : Outport
  wires:
  magic factor/1 -> Product/1
  Constant1/1 -> Relational Operator1/2
  Relational Operator/1 -> Logical Operator/2
  negative prc threshold/1 -> Relational Operator/2
  Relational Operator1/1 -> Logical Operator/1
  Logical Operator/1 -> Switch/2  "sig_BrakeOn"
  Max_Reku/1 -> Switch/1
  Switch/1 -> TargetRecuperation/1  "sig_TrqTargetRecup"
  Product/1 -> Switch/3  "sig_MaxRecTrqCoasting"
  km/h-->m/s/1 -> 1/R_Rad/1  "m_s"
  1/R_Rad/1 -> Product/2  "rad_s"
  vehicle mass [t]/1 -> magic factor/1
  rpm-->rad/s/1 -> Product/3
  BusIn/1 -> Bus Selector3/1  "ClutchSwTop_Rq"
  Bus Selector3/1 -> Relational Operator1/1  "<sig_BrakeOn_bool>"
  Bus Selector3/2 -> Relational Operator/1  "<sig_RetTorque_Nm>"
  Bus Selector3/4 -> rpm-->rad/s/1  "<sig_EngSpd_rpm>"
  Bus Selector3/3 -> km/h-->m/s/1  "<sig_VehSpd_kmh>"

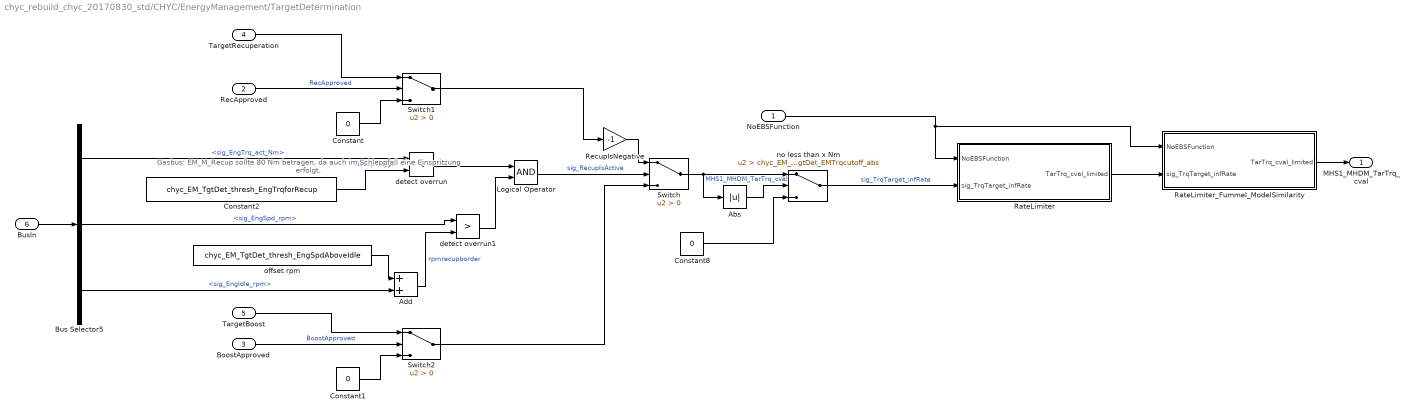
== system chyc_rebuild_chyc_20170830_std/CHYC/EnergyManagement/TargetDetermination ==
  note: Gasbus: EM_M_Recup sollte 80 Nm betragen, da auch im Schleppfall eine Einspritzung erfolgt.
  NoEBSFunction : Inport
  RecApproved : Inport  Port=2
  BoostApproved : Inport  Port=3
  TargetRecuperation : Inport  Port=4
  TargetBoost : Inport  Port=5
  BusIn : Inport  Port=6
  Abs : Abs
  Add : Sum
  Bus Selector5 : BusSelector  OutputSignals=sig_EngTrq_act_Nm,sig_EngSpd_rpm,sig_EngIdle_rpm
  Constant : Constant  Value=0
  Constant1 : Constant  Value=0
  Constant2 : Constant  Value=chyc_EM_TgtDet_thresh_EngTrqforRecup
  Constant8 : Constant  Value=0
  Logical Operator : Logic  AllPortsSameDT=off  OutDataTypeStr=boolean
  RateLimiter : Subsystem
  RateLimiter_Fummel_ModelSimilarity : Subsystem
  RecupIsNegative : Gain  Gain=-1
  Switch : Switch  Criteria=u2 > Threshold
  Switch1 : Switch  Criteria=u2 > Threshold
  Switch2 : Switch  Criteria=u2 > Threshold
  detect overrun : RelationalOperator  Operator=<  OutDataTypeStr=boolean
  detect overrun1 : RelationalOperator  Operator=>  OutDataTypeStr=boolean
  no less than x Nm : Switch  Criteria=u2 > Threshold  Threshold=chyc_EM_TgtDet_EMTrqcutoff_abs
  offset rpm : Constant  Value=chyc_EM_TgtDet_thresh_EngSpdAboveIdle
  MHS1_MHDM_TarTrq_cval : Outport
  wires:
  RateLimiter/1(TarTrq_cval_limited) -> RateLimiter_Fummel_ModelSimilarity/2(sig_TrqTarget_infRate)
  Abs/1 -> no less than x Nm/2
  Constant8/1 -> no less than x Nm/3
  Switch/1 -> no less than x Nm/1, Abs/1  "MHS1_MHDM_TarTrq_cval"
  RecApproved/1 -> Switch1/2  "RecApproved"
  BoostApproved/1 -> Switch2/2  "BoostApproved"
  Constant2/1 -> detect overrun/2  "RecupTrigger"
  TargetRecuperation/1 -> Switch1/1
  Constant/1 -> Switch1/3
  Switch1/1 -> RecupIsNegative/1
  TargetBoost/1 -> Switch2/1
  Constant1/1 -> Switch2/3
  Switch2/1 -> Switch/3
  detect overrun/1 -> Logical Operator/1
  detect overrun1/1 -> Logical Operator/2
  Add/1 -> detect overrun1/2  "rpmrecupborder"
  offset rpm/1 -> Add/1
  Logical Operator/1 -> Switch/2  "sig_RecupIsActive"
  RecupIsNegative/1 -> Switch/1
  Bus Selector5/1 -> detect overrun/1  "<sig_EngTrq_act_Nm>"
  Bus Selector5/2 -> detect overrun1/1  "<sig_EngSpd_rpm>"
  Bus Selector5/3 -> Add/2  "<sig_EngIdle_rpm>"
  BusIn/1 -> Bus Selector5/1
  NoEBSFunction/1 -> RateLimiter/1(NoEBSFunction), RateLimiter_Fummel_ModelSimilarity/1(NoEBSFunction)
  no less than x Nm/1 -> RateLimiter/2(sig_TrqTarget_infRate)  "sig_TrqTarget_infRate"
  RateLimiter_Fummel_ModelSimilarity/1(TarTrq_cval_limited) -> MHS1_MHDM_TarTrq_cval/1

== system chyc_rebuild_chyc_20170830_std/CHYC/MHSctrl/RKM_Ctrl  ==
  note: mit Logik für Recov / Boost
      | Recov:   RKM_C_S =
      | Boost:    RKM_C_S =
  M_EM_actual : Inport
  "U_ZK " : Inport  Port=2
  Logical Operator : Logic  AllPortsSameDT=off  OutDataTypeStr=boolean
  M_min : Constant  Value=0
  M_min1 : Constant  Value=51.8
  Relational Operator1 : RelationalOperator  Operator=>  OutDataTypeStr=boolean
  Relational Operator3 : RelationalOperator  Operator=<  OutDataTypeStr=boolean
  RKM_Control_Signal : Outport
  wires:
  Relational Operator3/1 -> Logical Operator/1
  Logical Operator/1 -> RKM_Control_Signal/1
  M_min/1 -> Relational Operator3/2
  M_min1/1 -> Relational Operator1/2
  "U_ZK "/1 -> Relational Operator1/1
  Relational Operator1/1 -> Logical Operator/2
  M_EM_actual/1 -> Relational Operator3/1

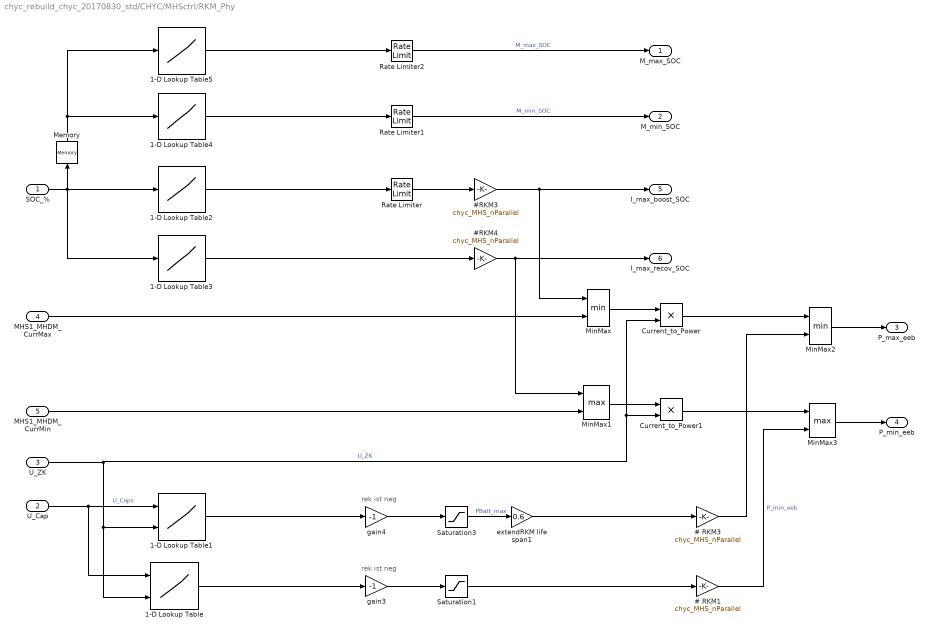
== system chyc_rebuild_chyc_20170830_std/CHYC/MHSctrl/RKM_Phy ==
  note: rek ist neg
  note: rek ist neg
  SOC_% : Inport
  U_Cap : Inport  Port=2
  U_ZK : Inport  Port=3
  MHS1_MHDM_CurrMax : Inport  Port=4
  MHS1_MHDM_CurrMin : Inport  Port=5
  # RKM1 : Gain  Gain=chyc_MHS_nParallel
  # RKM3 : Gain  Gain=chyc_MHS_nParallel
  #RKM3 : Gain  Gain=chyc_MHS_nParallel
  #RKM4 : Gain  Gain=chyc_MHS_nParallel
  1-D Lookup Table : Lookup_n-D  BreakpointsForDimension1=chyc_MHS_dcdc_U_Cap  BreakpointsForDimension2=chyc_MHS_dcdc_U_ZK  Table=chyc_MHS_dcdc_Pmax_chg  RndMeth=Simplest  InputSameDT=on
      settings: AttributesFormatString=%<Table>
  1-D Lookup Table1 : Lookup_n-D  BreakpointsForDimension1=chyc_MHS_dcdc_U_Cap  BreakpointsForDimension2=chyc_MHS_dcdc_U_ZK  Table=chyc_MHS_dcdc_Pmax_dischg  RndMeth=Simplest  InputSameDT=on
      settings: AttributesFormatString=%<Table>
  1-D Lookup Table2 : Lookup_n-D  NumberOfTableDimensions=1  BreakpointsForDimension1=[0,0.25,0.5,1,100]  Table=[0,20,80,200,200]  ExtrapMethod=Clip  UseLastTableValue=on  RndMeth=Simplest  InputSameDT=on
  1-D Lookup Table3 : Lookup_n-D  NumberOfTableDimensions=1  BreakpointsForDimension1=[0,99,99.5,99.75,100]  Table=[-200,-200,-80,-20,0]  ExtrapMethod=Clip  UseLastTableValue=on  RndMeth=Simplest  InputSameDT=on
  1-D Lookup Table4 : Lookup_n-D  NumberOfTableDimensions=1  BreakpointsForDimension1=[0,97,97.5,98,98.5,99,99.75,100]  Table=[-310,-310,-180,-50,-15,-5,-1,0]  ExtrapMethod=Clip  UseLastTableValue=on  RndMeth=Simplest  InputSameDT=on
  1-D Lookup Table5 : Lookup_n-D  NumberOfTableDimensions=1  BreakpointsForDimension1=[0,0.25,1,1.5,2,2.5,3,100]  Table=[0,1,5,15,50,180,310,310]  ExtrapMethod=Clip  UseLastTableValue=on  RndMeth=Simplest  InputSameDT=on
  Current_to_Power : Product  Inputs=**  RndMeth=Zero
  Current_to_Power1 : Product  Inputs=**  RndMeth=Zero
  Memory : Memory
  MinMax : MinMax  Inputs=2
  MinMax1 : MinMax  Function=max  Inputs=2
  MinMax2 : MinMax  Inputs=2
  MinMax3 : MinMax  Function=max  Inputs=2
  Rate Limiter : RateLimiter  RisingSlewLimit=200  FallingSlewLimit=-inf  SampleTimeMode=inherited
  Rate Limiter1 : RateLimiter  RisingSlewLimit=inf  FallingSlewLimit=-200  SampleTimeMode=inherited
  Rate Limiter2 : RateLimiter  RisingSlewLimit=200  FallingSlewLimit=-inf  SampleTimeMode=inherited
  Saturation1 : Saturate  UpperLimit=chyc_MHS_PEEBmax  LowerLimit=-chyc_MHS_PEEBmax
  Saturation3 : Saturate  UpperLimit=chyc_MHS_PEEBmax  LowerLimit=-chyc_MHS_PEEBmax
  extendRKM life span1 : Gain  Gain=0.6
  gain3 : Gain  Gain=-1
  gain4 : Gain  Gain=-1
  M_max_SOC : Outport
  M_min_SOC : Outport  Port=2
  P_max_eeb : Outport  Port=3
  P_min_eeb : Outport  Port=4
  I_max_boost_SOC : Outport  Port=5
  I_max_recov_SOC : Outport  Port=6
  wires:
  Memory/1 -> 1-D Lookup Table4/1, 1-D Lookup Table5/1
  1-D Lookup Table5/1 -> Rate Limiter2/1
  1-D Lookup Table4/1 -> Rate Limiter1/1
  Rate Limiter1/1 -> M_min_SOC/1  "M_min_SOC"
  Rate Limiter2/1 -> M_max_SOC/1  "M_max_SOC"
  1-D Lookup Table/1 -> gain3/1
  1-D Lookup Table1/1 -> gain4/1
  # RKM1/1 -> MinMax3/2  "P_min_eeb"
  # RKM3/1 -> MinMax2/2
  gain3/1 -> Saturation1/1
  gain4/1 -> Saturation3/1
  Saturation3/1 -> extendRKM life span1/1  "PBatt_max"
  1-D Lookup Table2/1 -> Rate Limiter/1
  U_ZK/1 -> Current_to_Power/2, Current_to_Power1/2, 1-D Lookup Table/2, 1-D Lookup Table1/2  "U_ZK"
  U_Cap/1 -> 1-D Lookup Table/1, 1-D Lookup Table1/1  "U_Caps"
  Rate Limiter/1 -> #RKM3/1
  #RKM3/1 -> MinMax/1, I_max_boost_SOC/1
  #RKM4/1 -> MinMax1/1, I_max_recov_SOC/1
  extendRKM life span1/1 -> # RKM3/1
  1-D Lookup Table3/1 -> #RKM4/1
  MHS1_MHDM_CurrMin/1 -> MinMax1/2
  SOC_%/1 -> Memory/1, 1-D Lookup Table3/1, 1-D Lookup Table2/1
  MHS1_MHDM_CurrMax/1 -> MinMax/2
  MinMax/1 -> Current_to_Power/1
  MinMax1/1 -> Current_to_Power1/1
  Current_to_Power/1 -> MinMax2/1
  Current_to_Power1/1 -> MinMax3/1
  MinMax2/1 -> P_max_eeb/1
  MinMax3/1 -> P_min_eeb/1
  Saturation1/1 -> # RKM1/1

== system chyc_rebuild_chyc_20170830_std/CHYC/MHSctrl/SOC ==
  note: SOC
  note: Ist_Energie
  note: Min_Energie
  note: E = 1/2 * C * (Umax^2 - Umin^2)
  U_Cap : Inport
  1/1 : Gain  Gain=1/2
  1/2 : Gain  Gain=1/2
  1/3 : Gain  Gain=1/2
  Add2 : Sum  Inputs=+-
  Add4 : Sum  Inputs=-+
  C : Gain  Gain=chyc_MHS_capacity
  "C " : Gain  Gain=chyc_MHS_capacity
  "C  " : Gain  Gain=chyc_MHS_capacity
  Divide1 : Product  Inputs=**
  Divide2 : Product  Inputs=**
  Divide3 : Product  Inputs=*/
  Divide4 : Product  Inputs=**
  U_cap_max : Constant  Value=chyc_MHS_U_cap_max
  U_cap_min : Constant  Value=chyc_MHS_U_cap_min
  SOC_RKM : Outport
  wires:
  U_Cap/1 -> Divide2/1, Divide2/2
  1/2/1 -> C/1
  Divide2/1 -> 1/2/1  "U_cap_quad"
  C/1 -> Add2/1
  1/1/1 -> "C "/1
  Divide1/1 -> 1/1/1  "U_cap_min_quad"
  U_cap_min/1 -> Divide1/2, Divide1/1
  "C "/1 -> Add2/2, Add4/1
  U_cap_max/1 -> Divide4/1, Divide4/2
  1/3/1 -> "C  "/1
  Divide4/1 -> 1/3/1  "U_cap_max_quad"
  "C  "/1 -> Add4/2
  Add2/1 -> Divide3/1  "E_delta_IST"
  Add4/1 -> Divide3/2  "E_delta_MAX"
  Divide3/1 -> SOC_RKM/1  "SOC_RKM"

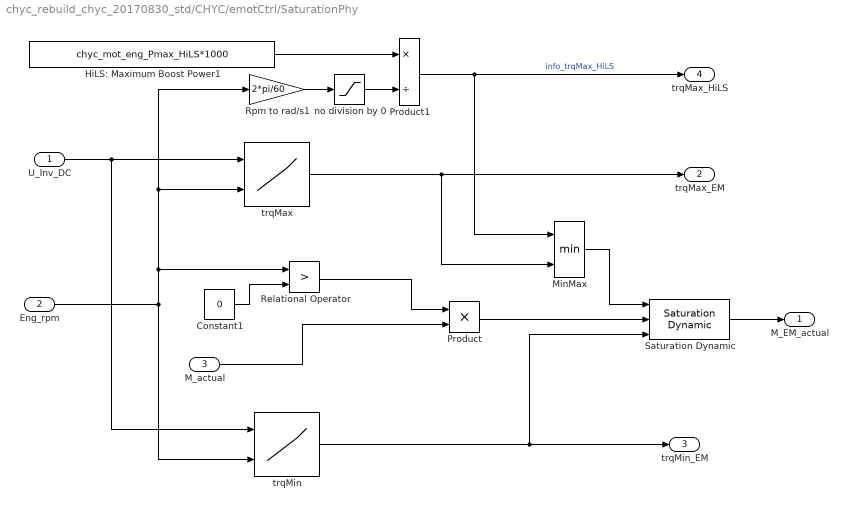
== system chyc_rebuild_chyc_20170830_std/CHYC/emotCtrl/SaturationPhy ==
  U_Inv_DC : Inport
  Eng_rpm : Inport  Port=2
  M_actual : Inport  Port=3
  Constant1 : Constant  Value=0
  HiLS: Maximum Boost Power1 : Constant  Value=chyc_mot_eng_Pmax_HiLS*1000
  MinMax : MinMax  Inputs=2
  Product : Product  RndMeth=Zero
  Product1 : Product  Inputs=*/  RndMeth=Zero
  Relational Operator : RelationalOperator  Operator=>  OutDataTypeStr=boolean
  Rpm to rad/s1 : Gain  Gain=2*pi/60
  Saturation Dynamic : simulink/Discontinuities/Saturation Dynamic  OutMin=[]  OutMax=[]  OutDataTypeStr=Inherit: Same as second input  OutDataType=fixdt(1, 16)  OutScaling=2^-10  DoSatur=off
  no division by 0 : Saturate  UpperLimit=inf  LowerLimit=10
  trqMax : Lookup_n-D  BreakpointsForDimension1=chyc_mot_trqMax_vltTab  BreakpointsForDimension2=chyc_mot_trqMax_nTab  BreakpointsForDimension3=[5, 7]  Table=chyc_mot_trqMax_trqTab_peak  RndMeth=Simplest  InputSameDT=on
  trqMin : Lookup_n-D  BreakpointsForDimension1=chyc_mot_trqMin_vltTab  BreakpointsForDimension2=chyc_mot_trqMin_nTab  BreakpointsForDimension3=[5, 7]  Table=chyc_mot_trqMin_trqTab_peak  RndMeth=Simplest  InputSameDT=on
  M_EM_actual : Outport
  trqMax_EM : Outport  Port=2
  trqMin_EM : Outport  Port=3
  trqMax_HiLS : Outport  Port=4
  wires:
  Constant1/1 -> Relational Operator/2
  Relational Operator/1 -> Product/1
  M_actual/1 -> Product/2
  Saturation Dynamic/1 -> M_EM_actual/1
  trqMin/1 -> trqMin_EM/1, Saturation Dynamic/3
  trqMax/1 -> trqMax_EM/1, MinMax/2
  Eng_rpm/1 -> trqMin/2, Rpm to rad/s1/1, trqMax/2, Relational Operator/1
  Product/1 -> Saturation Dynamic/2
  Product1/1 -> trqMax_HiLS/1, MinMax/1  "info_trqMax_HiLS"
  Rpm to rad/s1/1 -> no division by 0/1
  HiLS: Maximum Boost Power1/1 -> Product1/1
  MinMax/1 -> Saturation Dynamic/1
  U_Inv_DC/1 -> trqMin/1, trqMax/1
  no division by 0/1 -> Product1/2

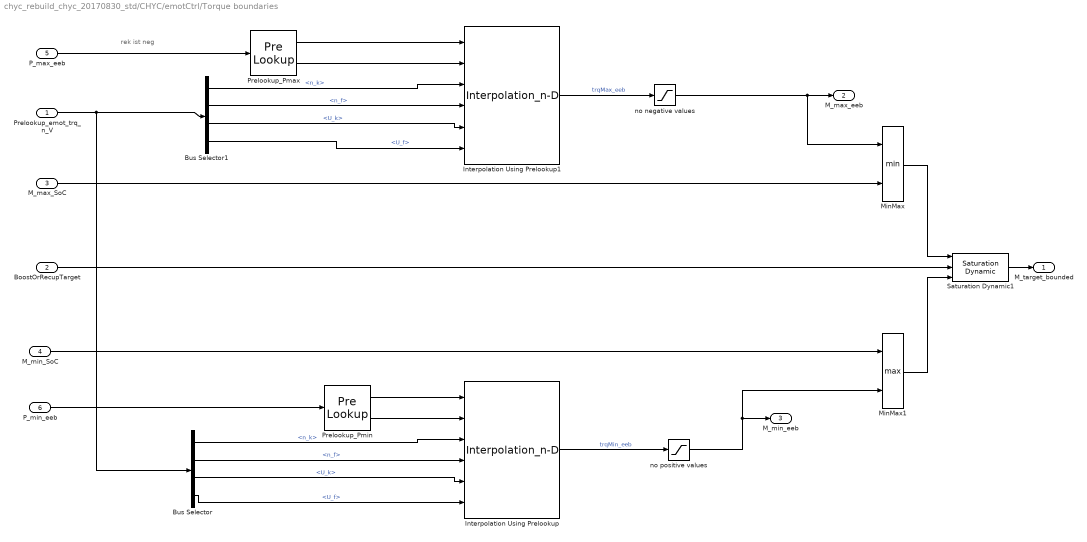
== system chyc_rebuild_chyc_20170830_std/CHYC/emotCtrl/Torque boundaries ==
  note: rek ist neg
  Prelookup_emot_trq_n_V : Inport
  BoostOrRecupTarget : Inport  Port=2
  M_max_SoC : Inport  Port=3
  M_min_SoC : Inport  Port=4
  P_max_eeb : Inport  Port=5
  P_min_eeb : Inport  Port=6
  Bus Selector : BusSelector  OutputSignals=n_k,n_f,U_k,U_f
  Bus Selector1 : BusSelector  OutputSignals=n_k,n_f,U_k,U_f
  Interpolation Using Prelookup : Interpolation_n-D  NumberOfTableDimensions=3  Table=chyc_mot_Pmax_PTab_trqTab
      settings: InputPortMap=u0,u1,u2,u3,u4,u5
  Interpolation Using Prelookup1 : Interpolation_n-D  NumberOfTableDimensions=3  Table=chyc_mot_Pmax_PTab_trqTab
      settings: InputPortMap=u0,u1,u2,u3,u4,u5
  MinMax : MinMax  Inputs=2
  MinMax1 : MinMax  Function=max  Inputs=2
  Prelookup_Pmax : PreLookup  BreakpointsData=chyc_mot_Pmax_PTab  IndexSearchMethod=Linear search  BeginIndexSearchUsingPreviousIndexResult=on  ExtrapMethod=Linear
  Prelookup_Pmin : PreLookup  BreakpointsData=chyc_mot_Pmax_PTab  IndexSearchMethod=Linear search  BeginIndexSearchUsingPreviousIndexResult=on  ExtrapMethod=Linear
  Saturation Dynamic1 : simulink/Discontinuities/Saturation Dynamic  OutMin=[]  OutMax=[]  OutDataTypeStr=Inherit: Same as second input  OutDataType=fixdt(1, 16)  OutScaling=2^-10  DoSatur=off
  no negative values : Saturate  UpperLimit=inf  LowerLimit=0
  no positive values : Saturate  UpperLimit=0  LowerLimit=-inf
  M_target_bounded : Outport
  M_max_eeb : Outport  Port=2
  M_min_eeb : Outport  Port=3
  wires:
  Interpolation Using Prelookup/1 -> no positive values/1  "trqMin_eeb"
  Interpolation Using Prelookup1/1 -> no negative values/1  "trqMax_eeb"
  Prelookup_emot_trq_n_V/1 -> Bus Selector/1, Bus Selector1/1
  Saturation Dynamic1/1 -> M_target_bounded/1
  BoostOrRecupTarget/1 -> Saturation Dynamic1/2
  MinMax/1 -> Saturation Dynamic1/1
  MinMax1/1 -> Saturation Dynamic1/3
  M_max_SoC/1 -> MinMax/2
  M_min_SoC/1 -> MinMax1/1
  P_min_eeb/1 -> Prelookup_Pmin/1
  Prelookup_Pmin/1 -> Interpolation Using Prelookup/1
  Prelookup_Pmin/2 -> Interpolation Using Prelookup/2
  P_max_eeb/1 -> Prelookup_Pmax/1
  Prelookup_Pmax/1 -> Interpolation Using Prelookup1/1
  Prelookup_Pmax/2 -> Interpolation Using Prelookup1/2
  Bus Selector/2 -> Interpolation Using Prelookup/4  "<n_f>"
  Bus Selector/3 -> Interpolation Using Prelookup/5  "<U_k>"
  Bus Selector/1 -> Interpolation Using Prelookup/3  "<n_k>"
  Bus Selector/4 -> Interpolation Using Prelookup/6  "<U_f>"
  Bus Selector1/1 -> Interpolation Using Prelookup1/3  "<n_k>"
  Bus Selector1/2 -> Interpolation Using Prelookup1/4  "<n_f>"
  Bus Selector1/3 -> Interpolation Using Prelookup1/5  "<U_k>"
  Bus Selector1/4 -> Interpolation Using Prelookup1/6  "<U_f>"
  no negative values/1 -> MinMax/1, M_max_eeb/1
  no positive values/1 -> MinMax1/2, M_min_eeb/1

== system chyc_rebuild_chyc_20170830_std/CHYC/emotCtrl/emotCtrl_voltage_control ==
  U_inv : Inport
  M_EM_target : Inport  Port=2
  U_req : Inport  Port=3
  Terminator : Terminator
  Terminator1 : Terminator
  M_actual : Outport
  wires:
  U_inv/1 -> Terminator1/1
  U_req/1 -> Terminator/1
  M_EM_target/1 -> M_actual/1  "M_actual"

== system chyc_rebuild_chyc_20170830_std/CHYC/emotCtrl/emot_Prelookup and el. Current ==
  nEmot : Inport
  U_inv_DC : Inport  Port=2
  trqEmot : Inport  Port=3
  Bus Creator : BusCreator  Inputs=6
  Prelookup_U_inv_DC : PreLookup  BreakpointsData=chyc_mot_vltTab  IndexSearchMethod=Linear search  BeginIndexSearchUsingPreviousIndexResult=on  ExtrapMethod=Linear  BreakpointDataTypeStr=Inherit: Inherit from 'Breakpoint data'  FractionDataTypeStr=double
      settings: LockScale=on
  Prelookup_nEmot : PreLookup  BreakpointsData=chyc_mot_nTab  IndexSearchMethod=Linear search  BeginIndexSearchUsingPreviousIndexResult=on  ExtrapMethod=Linear  BreakpointDataTypeStr=Inherit: Inherit from 'Breakpoint data'  FractionDataTypeStr=double
      settings: LockScale=on
  Prelookup_trqEmot : PreLookup  BreakpointsData=chyc_mot_trqTab  IndexSearchMethod=Linear search  BeginIndexSearchUsingPreviousIndexResult=on  ExtrapMethod=Linear  BreakpointDataTypeStr=Inherit: Inherit from 'Breakpoint data'  FractionDataTypeStr=double
  Prelookup_emot_trq_n_U : Outport
  wires:
  Prelookup_U_inv_DC/1 -> Bus Creator/5  "U_k"
  Prelookup_U_inv_DC/2 -> Bus Creator/6  "U_f"
  Prelookup_nEmot/2 -> Bus Creator/4  "n_f"
  U_inv_DC/1 -> Prelookup_U_inv_DC/1
  Prelookup_nEmot/1 -> Bus Creator/3  "n_k"
  Prelookup_trqEmot/1 -> Bus Creator/1  "trq_k"
  trqEmot/1 -> Prelookup_trqEmot/1
  Prelookup_trqEmot/2 -> Bus Creator/2  "trq_f"
  nEmot/1 -> Prelookup_nEmot/1
  Bus Creator/1 -> Prelookup_emot_trq_n_U/1

== system chyc_rebuild_chyc_20170830_std/CHYC/EnergyManagement/TargetDetermination/RateLimiter ==
  NoEBSFunction : Inport
  sig_TrqTarget_infRate : Inport  Port=2
  Constant3 : Constant  Value=0
  Constant4 : Constant  Value=chyc_EM_TgtDet_trqRateLimit_EBS_activate_pos
  Constant5 : Constant  Value=chyc_EM_TgtDet_trqRateLimit_boost
  Constant6 : Constant  Value=chyc_EM_TgtDet_trqRateLimit_EBS_activate_neg
  Constant7 : Constant  Value=chyc_EM_TgtDet_trqRateLimit_recup
  Rate Limiter Dynamic : simulink/Discontinuities/Rate Limiter Dynamic
  Switch3 : Switch  Criteria=u2 > Threshold
  Switch4 : Switch  Criteria=u2 > Threshold
  Switch5 : Switch  Criteria=u2 > Threshold
  TarTrq_cval_limited : Outport
  wires:
  Rate Limiter Dynamic/1 -> TarTrq_cval_limited/1  "MHS1_MHDM_TarTrq_cval"
  Constant3/1 -> Switch3/3
  NoEBSFunction/1 -> Switch4/2, Switch5/2, Switch3/2
  Constant4/1 -> Switch5/3
  Constant6/1 -> Switch4/3
  Switch5/1 -> Rate Limiter Dynamic/1
  Switch4/1 -> Rate Limiter Dynamic/3
  Switch3/1 -> Rate Limiter Dynamic/2  "sig_TrqTarget_infRate"
  Constant5/1 -> Switch5/1
  sig_TrqTarget_infRate/1 -> Switch3/1
  Constant7/1 -> Switch4/1

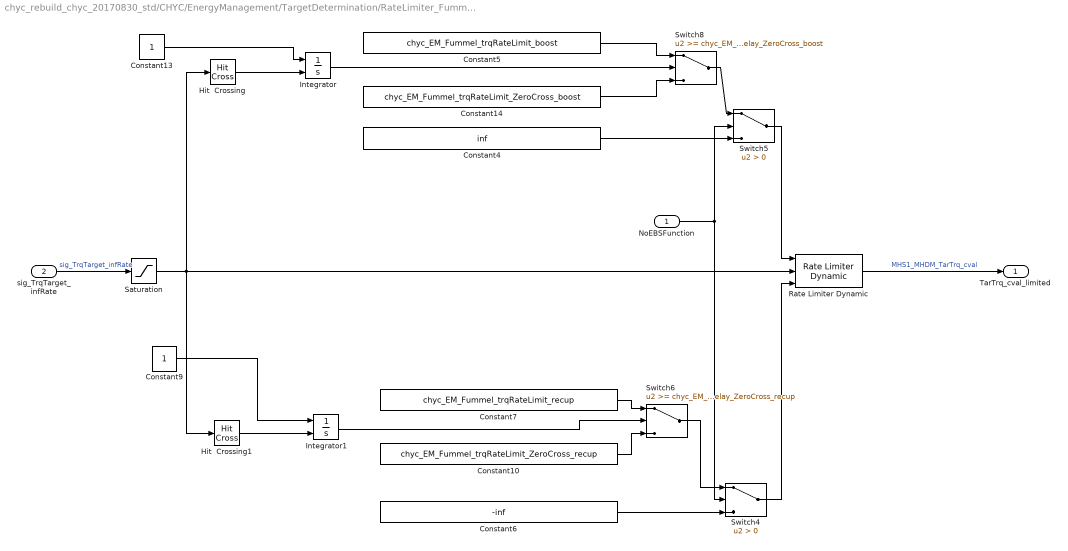
== system chyc_rebuild_chyc_20170830_std/CHYC/EnergyManagement/TargetDetermination/RateLimiter_Fummel_ModelSimilarity ==
  NoEBSFunction : Inport
  sig_TrqTarget_infRate : Inport  Port=2
  Constant10 : Constant  Value=chyc_EM_Fummel_trqRateLimit_ZeroCross_recup
  Constant13 : Constant
  Constant14 : Constant  Value=chyc_EM_Fummel_trqRateLimit_ZeroCross_boost
  Constant4 : Constant  Value=inf
  Constant5 : Constant  Value=chyc_EM_Fummel_trqRateLimit_boost
  Constant6 : Constant  Value=-inf
  Constant7 : Constant  Value=chyc_EM_Fummel_trqRateLimit_recup
  Constant9 : Constant
  Hit  Crossing : HitCross  HitCrossingOffset=chyc_EM_Fummel_trqThreshold_ZeroCross_boost  HitCrossingDirection=rising
  Hit  Crossing1 : HitCross  HitCrossingOffset=chyc_EM_Fummel_trqThreshold_ZeroCross_recup  HitCrossingDirection=falling
  Integrator : Integrator  ExternalReset=rising
  Integrator1 : Integrator  ExternalReset=rising  LimitOutput=on  UpperSaturationLimit=100  LowerSaturationLimit=0
  Rate Limiter Dynamic : simulink/Discontinuities/Rate Limiter Dynamic
  Saturation : Saturate  UpperLimit=chyc_EM_Fummel_TrqTargetLimit_boost  LowerLimit=chyc_EM_Fummel_TrqTargetLimit_recup
  Switch4 : Switch  Criteria=u2 > Threshold
  Switch5 : Switch  Criteria=u2 > Threshold
  Switch6 : Switch  Threshold=chyc_EM_Fummel_rateDelay_ZeroCross_recup
  Switch8 : Switch  Threshold=chyc_EM_Fummel_rateDelay_ZeroCross_boost
  TarTrq_cval_limited : Outport
  wires:
  Saturation/1 -> Hit  Crossing/1, Rate Limiter Dynamic/2, Hit  Crossing1/1
  Switch6/1 -> Switch4/1
  Constant9/1 -> Integrator1/1
  Integrator1/1 -> Switch6/2
  Hit  Crossing1/1 -> Integrator1/2
  Constant10/1 -> Switch6/3
  Hit  Crossing/1 -> Integrator/2
  Switch8/1 -> Switch5/1
  Constant14/1 -> Switch8/3
  sig_TrqTarget_infRate/1 -> Saturation/1  "sig_TrqTarget_infRate"
  Integrator/1 -> Switch8/2
  Constant13/1 -> Integrator/1
  Switch4/1 -> Rate Limiter Dynamic/3
  Switch5/1 -> Rate Limiter Dynamic/1
  Constant6/1 -> Switch4/3
  Constant7/1 -> Switch6/1
  Constant5/1 -> Switch8/1
  Constant4/1 -> Switch5/3
  NoEBSFunction/1 -> Switch4/2, Switch5/2
  Rate Limiter Dynamic/1 -> TarTrq_cval_limited/1  "MHS1_MHDM_TarTrq_cval"
